simulink model "SM_CirRLC"  (R2023b)
settings: Solver=ode23  StartTime=0.0  StopTime=0.0005  RelTol=1e-3
values from neighbouring files (symbols this model uses):
  c = 0.1e-6    (= 1e-07)    [CirRLC.m]    (also in RLC.mat; Rlc.mat)
  l = 4e-3    (= 0.004)    [CirRLC.m]    (also in RLC.mat; Rlc.mat)
  r = 120    [CirRLC.m]    (also in RLC.mat = 100; Rlc.mat)

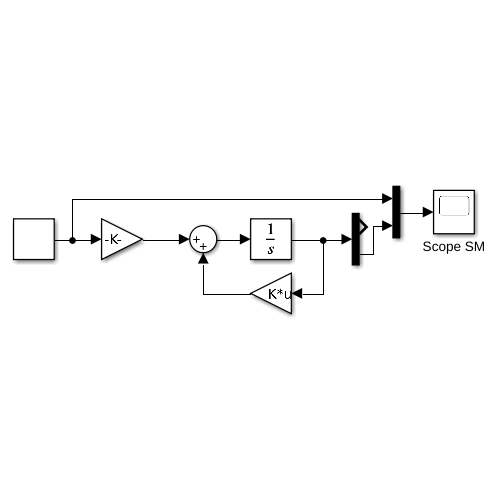
[thumbnail: Simulink's stored preview of the top-level diagram]
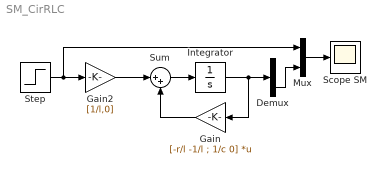
== system SM_CirRLC ==
  Demux : Demux  Outputs=2
  Gain : Gain  Gain=[-r/l -1/l ; 1/c 0]  Multiplication=Matrix(K*u)
  Gain2 : Gain  Gain=[1/l,0]
  Integrator : Integrator
  Mux : Mux  Inputs=2
  Scope SM : Scope
  Step : Step  Time=0  After=12  SampleTime=0
  Sum : Sum  Inputs=|++
  wires:
  Integrator/1 -> Gain/1, Demux/1
  Sum/1 -> Integrator/1
  Gain2/1 -> Sum/1
  Mux/1 -> Scope SM/1
  Step/1 -> Mux/1, Gain2/1
  Gain/1 -> Sum/2
  Demux/2 -> Mux/2
